simulink model "MRAC_Augmented_Error_Solution_Known_control_gain"  (R2023b)
settings: Solver=FixedStepAuto  StartTime=0.0  StopTime=200  FixedStep=1e-3  RelTol=1e-3
values from neighbouring files (symbols this model uses):
  a0 = 6    [value_tuning.m]
  a1 = 7    [value_tuning.m]
  b0 = 6    [value_tuning.m]
  b_min = 0.1    [value_tuning.m]
  gamma = 0.05    [value_tuning.m]
  k0 = 3    [value_tuning.m]
  k_M0 = 1    [value_tuning.m]
  k_M1 = 2    [value_tuning.m]
settings Model: Creator=nguye  LastModifiedBy=nguye

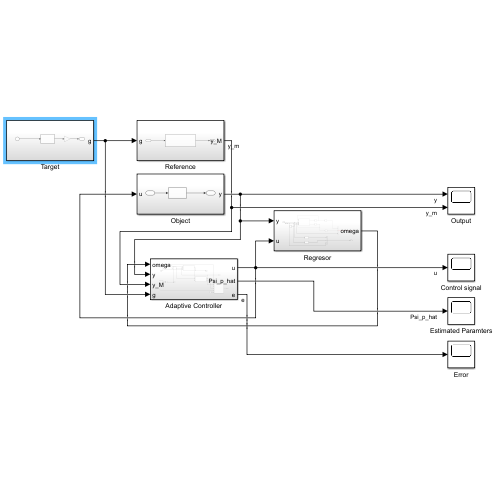
[thumbnail: Simulink's stored preview of the top-level diagram]
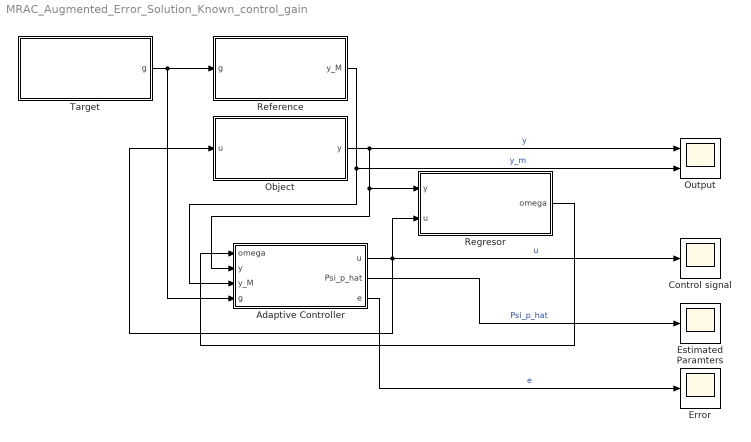
== system MRAC_Augmented_Error_Solution_Known_control_gain ==
  Adaptive Controller : Subsystem
  Control signal : Scope
  Error : Scope
  Estimated Paramters : Scope
  Object : Subsystem
  Output : Scope  NumInputPorts=2
  Reference : Subsystem
  Regresor : Subsystem
  Target : Subsystem
  wires:
  Object/1(y) -> Adaptive Controller/2(y), Regresor/1(y), Output/1  "y"
  Adaptive Controller/1(u) -> Regresor/2(u), Control signal/1, Object/1(u)  "u"
  Target/1(g) -> Adaptive Controller/4(g), Reference/1(g)
  Regresor/1(omega) -> Adaptive Controller/1(omega)
  Reference/1(y_M) -> Output/2, Adaptive Controller/3(y_M)  "y_m"
  Adaptive Controller/2(Psi_p_hat) -> Estimated Paramters/1  "Psi_p_hat"
  Adaptive Controller/3(e) -> Error/1  "e"

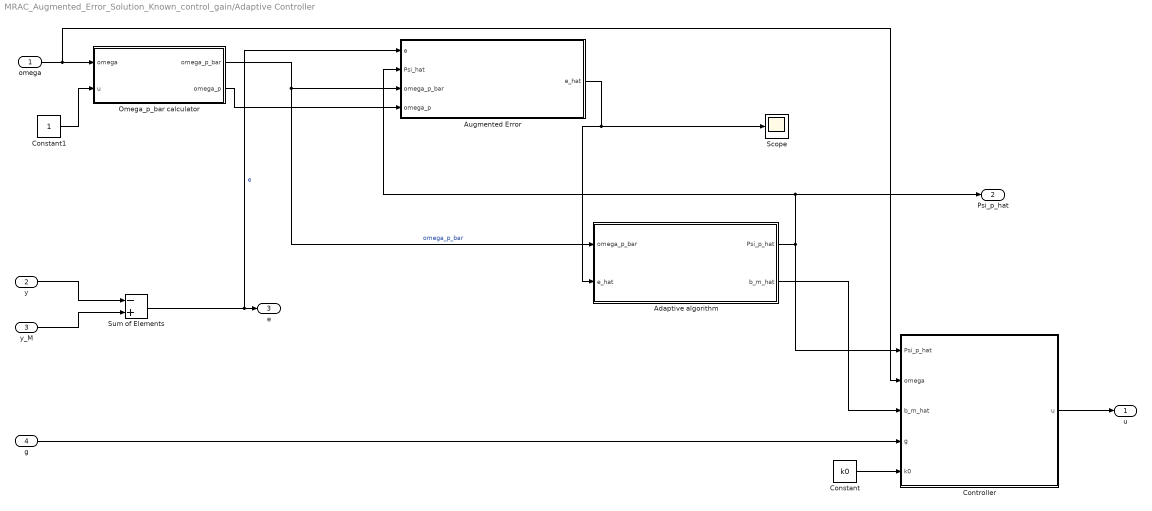
== system MRAC_Augmented_Error_Solution_Known_control_gain/Adaptive Controller ==
  omega : Inport
  y : Inport  Port=2
  y_M : Inport  Port=3
  g : Inport  Port=4
  Adaptive algorithm : Subsystem
  Augmented Error : Subsystem
  Constant : Constant  Value=k0
  Constant1 : Constant
  Controller : MATLAB Function  TreatAsAtomicUnit=on
  Omega_p_bar calculator : Subsystem
  Scope : Scope
  Sum of Elements : Sum  Inputs=-+
  u : Outport
  Psi_p_hat : Outport  Port=2
  e : Outport  Port=3
  wires:
  omega/1 -> Controller/2(omega), Omega_p_bar calculator/1(omega)
  y_M/1 -> Sum of Elements/2
  y/1 -> Sum of Elements/1
  Sum of Elements/1 -> e/1, Augmented Error/1(e)  "e"
  Omega_p_bar calculator/1(omega_p_bar) -> Adaptive algorithm/1(omega_p_bar), Augmented Error/3(omega_p_bar)  "omega_p_bar"
  Adaptive algorithm/1(Psi_p_hat) -> Controller/1(Psi_p_hat), Psi_p_hat/1, Augmented Error/2(Psi_hat)
  Controller/1(u) -> u/1
  g/1 -> Controller/4(g)
  Constant/1 -> Controller/5(k0)
  Augmented Error/1(e_hat) -> Adaptive algorithm/2(e_hat), Scope/1
  Adaptive algorithm/2(b_m_hat) -> Controller/3(b_m_hat)
  Omega_p_bar calculator/2(omega_p) -> Augmented Error/4(omega_p)
  Constant1/1 -> Omega_p_bar calculator/2(u)

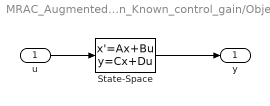
== system MRAC_Augmented_Error_Solution_Known_control_gain/Object ==
  u : Inport
  State-Space : StateSpace  A=[0, 1; -a0, -a1]  B=[0; b0]  C=[1, 0]  D=0  InitialCondition=1
  y : Outport
  wires:
  u/1 -> State-Space/1
  State-Space/1 -> y/1

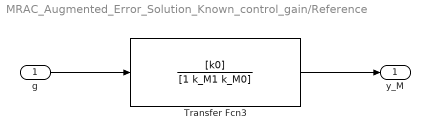
== system MRAC_Augmented_Error_Solution_Known_control_gain/Reference ==
  g : Inport
  Transfer Fcn3 : TransferFcn  Numerator=[k0]  Denominator=[1 k_M1 k_M0]
  y_M : Outport
  wires:
  g/1 -> Transfer Fcn3/1
  Transfer Fcn3/1 -> y_M/1

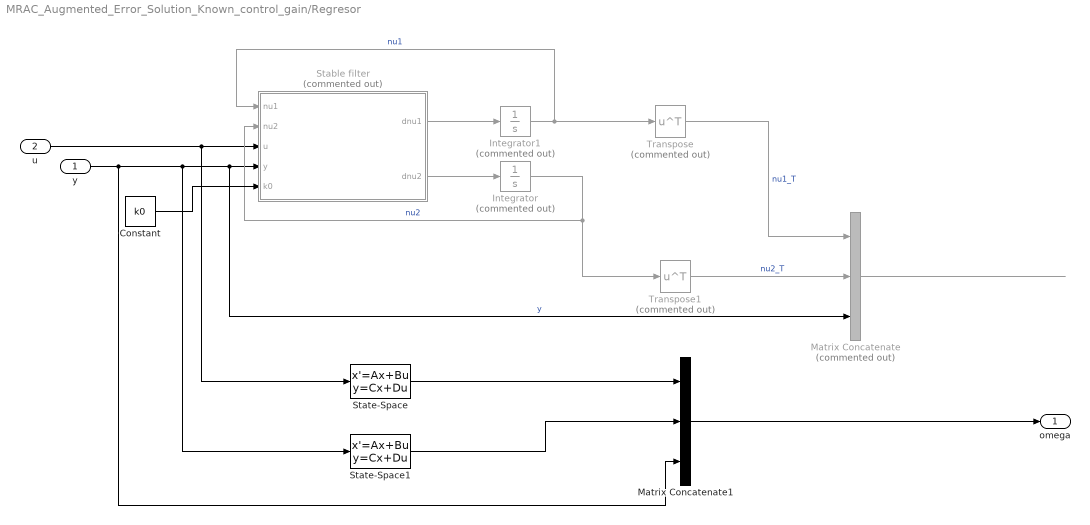
== system MRAC_Augmented_Error_Solution_Known_control_gain/Regresor ==
  y : Inport
  u : Inport  Port=2
  Constant : Constant  Value=k0
  Integrator : Integrator  Commented=on
  Integrator1 : Integrator  Commented=on
  Matrix Concatenate : Concatenate  Commented=on  NumInputs=3  ConcatenateDimension=2
  Matrix Concatenate1 : Concatenate  NumInputs=3  ConcatenateDimension=2
  Stable filter : MATLAB Function  Commented=on  TreatAsAtomicUnit=on
  State-Space : StateSpace  A=-k0  InitialCondition=0
  State-Space1 : StateSpace  A=-k0  InitialCondition=0
  Transpose : Math  Commented=on  Operator=transpose
  Transpose1 : Math  Commented=on  Operator=transpose
  omega : Outport
  wires:
  u/1 -> State-Space/1, Stable filter/3(u)
  y/1 -> Matrix Concatenate1/3, State-Space1/1, Matrix Concatenate/3, Stable filter/4(y)  "y"
  Stable filter/2(dnu2) -> Integrator/1
  Stable filter/1(dnu1) -> Integrator1/1
  Integrator1/1 -> Transpose/1, Stable filter/1(nu1)  "nu1"
  Integrator/1 -> Transpose1/1, Stable filter/2(nu2)  "nu2"
  Matrix Concatenate/1 -> ?
  Transpose/1 -> Matrix Concatenate/1  "nu1_T"
  Transpose1/1 -> Matrix Concatenate/2  "nu2_T"
  Constant/1 -> Stable filter/5(k0)
  State-Space1/1 -> Matrix Concatenate1/2
  State-Space/1 -> Matrix Concatenate1/1
  Matrix Concatenate1/1 -> omega/1

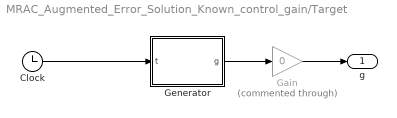
== system MRAC_Augmented_Error_Solution_Known_control_gain/Target ==
  Clock : Clock
  Gain : Gain  Commented=through  Gain=0
  Generator : MATLAB Function  TreatAsAtomicUnit=on
  g : Outport
  wires:
  Generator/1(g) -> Gain/1
  Clock/1 -> Generator/1(t)
  Gain/1 -> g/1

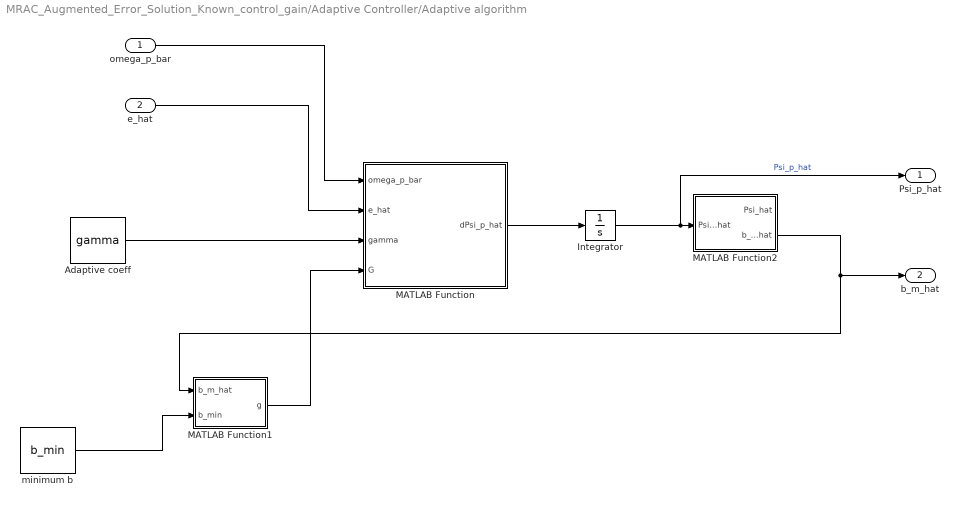
== system MRAC_Augmented_Error_Solution_Known_control_gain/Adaptive Controller/Adaptive algorithm ==
  omega_p_bar : Inport
  e_hat : Inport  Port=2
  Adaptive coeff : Constant  Value=gamma
  Integrator : Integrator  InitialCondition=1
  MATLAB Function : MATLAB Function  TreatAsAtomicUnit=on
  MATLAB Function1 : MATLAB Function  TreatAsAtomicUnit=on
  MATLAB Function2 : MATLAB Function  TreatAsAtomicUnit=on
  minimum b : Constant  Value=b_min
  Psi_p_hat : Outport
  b_m_hat : Outport  Port=2
  wires:
  omega_p_bar/1 -> MATLAB Function/1(omega_p_bar)
  e_hat/1 -> MATLAB Function/2(e_hat)
  MATLAB Function/1(dPsi_p_hat) -> Integrator/1
  Adaptive coeff/1 -> MATLAB Function/3(gamma)
  minimum b/1 -> MATLAB Function1/2(b_min)
  MATLAB Function1/1(g) -> MATLAB Function/4(G)
  Integrator/1 -> Psi_p_hat/1, MATLAB Function2/1(Psi_p_hat)  "Psi_p_hat"
  MATLAB Function2/2(b_m_hat) -> MATLAB Function1/1(b_m_hat), b_m_hat/1

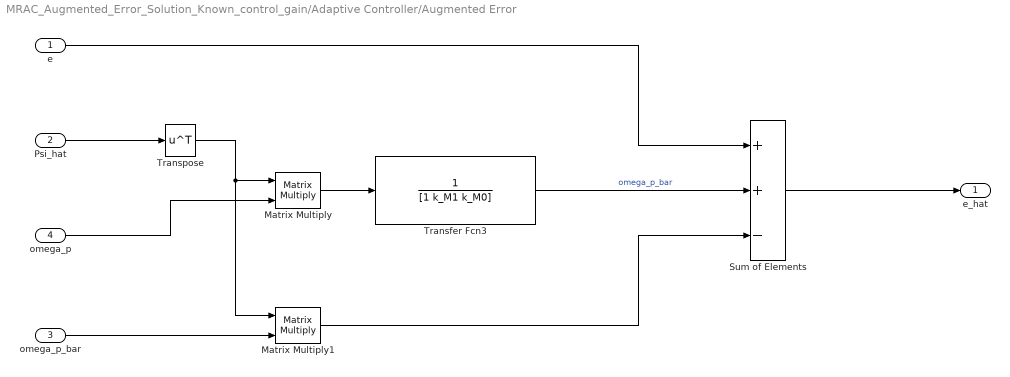
== system MRAC_Augmented_Error_Solution_Known_control_gain/Adaptive Controller/Augmented Error ==
  e : Inport
  Psi_hat : Inport  Port=2
  omega_p_bar : Inport  Port=3
  omega_p : Inport  Port=4
  Matrix Multiply : Product  Multiplication=Matrix(*)
  Matrix Multiply1 : Product  Multiplication=Matrix(*)
  Sum of Elements : Sum  Inputs=++-
  Transfer Fcn3 : TransferFcn  Denominator=[1 k_M1 k_M0]
  Transpose : Math  Operator=transpose
  e_hat : Outport
  wires:
  Psi_hat/1 -> Transpose/1
  omega_p/1 -> Matrix Multiply/2
  Transpose/1 -> Matrix Multiply1/1, Matrix Multiply/1
  Matrix Multiply/1 -> Transfer Fcn3/1
  omega_p_bar/1 -> Matrix Multiply1/2
  e/1 -> Sum of Elements/1
  Matrix Multiply1/1 -> Sum of Elements/3
  Transfer Fcn3/1 -> Sum of Elements/2  "omega_p_bar"
  Sum of Elements/1 -> e_hat/1

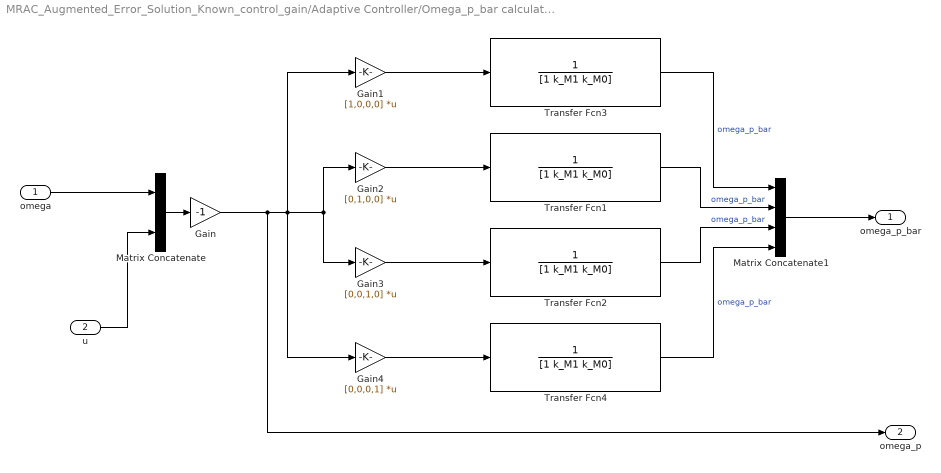
== system MRAC_Augmented_Error_Solution_Known_control_gain/Adaptive Controller/Omega_p_bar calculator ==
  omega : Inport
  u : Inport  Port=2
  Gain : Gain  Gain=-1
  Gain1 : Gain  Gain=[1,0,0,0]  Multiplication=Matrix(K*u)
  Gain2 : Gain  Gain=[0,1,0,0]  Multiplication=Matrix(K*u)
  Gain3 : Gain  Gain=[0,0,1,0]  Multiplication=Matrix(K*u)
  Gain4 : Gain  Gain=[0,0,0,1]  Multiplication=Matrix(K*u)
  Matrix Concatenate : Concatenate  ConcatenateDimension=2
  Matrix Concatenate1 : Concatenate  NumInputs=4  ConcatenateDimension=2
  Transfer Fcn{1..4} (4 alike) : TransferFcn  Denominator=[1 k_M1 k_M0]
  omega_p_bar : Outport
  omega_p : Outport  Port=2
  wires:
  Gain/1 -> omega_p/1, Gain1/1, Gain2/1, Gain3/1, Gain4/1
  Transfer Fcn1/1 -> Matrix Concatenate1/2  "omega_p_bar"
  Transfer Fcn3/1 -> Matrix Concatenate1/1  "omega_p_bar"
  Transfer Fcn2/1 -> Matrix Concatenate1/3  "omega_p_bar"
  Matrix Concatenate1/1 -> omega_p_bar/1
  u/1 -> Matrix Concatenate/2
  Matrix Concatenate/1 -> Gain/1
  Transfer Fcn4/1 -> Matrix Concatenate1/4  "omega_p_bar"
  omega/1 -> Matrix Concatenate/1
  Gain1/1 -> Transfer Fcn3/1
  Gain2/1 -> Transfer Fcn1/1
  Gain3/1 -> Transfer Fcn2/1
  Gain4/1 -> Transfer Fcn4/1

== matlab function MRAC_Augmented_Error_Solution_Known_control_gain/Target/Generator ==
  data: t input; g output
function g = fcn(t)

g = 3*sign(sin(0.5*t));

== matlab function MRAC_Augmented_Error_Solution_Known_control_gain/Regresor/Stable filter ==
  data: nu1 input; nu2 input; u input; dnu1 output; y input; dnu2 output; k0 input
function [dnu1, dnu2] = fcn(nu1, nu2, u, y, k0)
%
% Stable filters in Lemma (R. V. Monopoli, 1974, direct control parameterization lemma )
%

%
Lambda = -k0;
dnu1 = Lambda*nu1 + u; 
dnu2 = Lambda*nu2 + y;

== matlab function MRAC_Augmented_Error_Solution_Known_control_gain/Adaptive Controller/Adaptive algorithm/MATLAB Function ==
  data: omega_p_bar input; dPsi_p_hat output; e_hat input; gamma input; G input
function dPsi_p_hat = fcn(omega_p_bar, e_hat, gamma, G)

dPsi_p_hat = gamma * G * omega_p_bar * e_hat / (1 + omega_p_bar'*omega_p_bar);

== matlab function MRAC_Augmented_Error_Solution_Known_control_gain/Adaptive Controller/Controller ==
  data: Psi_p_hat input; u output; omega input; b_m_hat input; g input; k0 input
function u = fcn(Psi_p_hat, omega, b_m_hat, g, k0)

u = 1/b_m_hat * (-Psi_p_hat(1:3)'*omega + k0*g);

== matlab function MRAC_Augmented_Error_Solution_Known_control_gain/Adaptive Controller/Adaptive algorithm/MATLAB Function1 ==
  data: b_m_hat input; g output; b_min input
function g = fcn(b_m_hat, b_min)
g=0;
if b_m_hat >= b_min
    g = eye(1);
elseif b_m_hat < b_min
    xi_2n = [0,1];
    g = eye(1) - xi_2n*xi_2n';
end

== matlab function MRAC_Augmented_Error_Solution_Known_control_gain/Adaptive Controller/Adaptive algorithm/MATLAB Function2 ==
  data: Psi_p_hat input; Psi_hat output; b_m_hat output
function [Psi_hat, b_m_hat]= fcn(Psi_p_hat)

Psi_hat = Psi_p_hat(1:2);
b_m_hat = Psi_p_hat(3);
